simulink subsystem "IMUSensor"  (R2023b)
settings: Solver=VariableStepAuto  StartTime=0.0  StopTime=10.0  RelTol=1e-3
libraries: vehdynlibsens x1
settings Model: Creator=The MathWorks, Inc.  LastModifiedBy=The MathWorks, Inc.

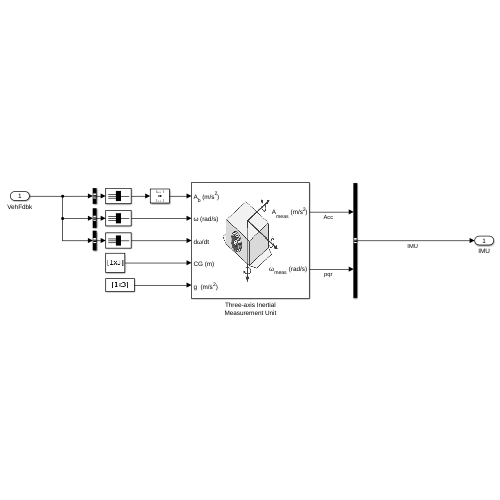
[thumbnail: Simulink's stored preview of the top-level diagram]
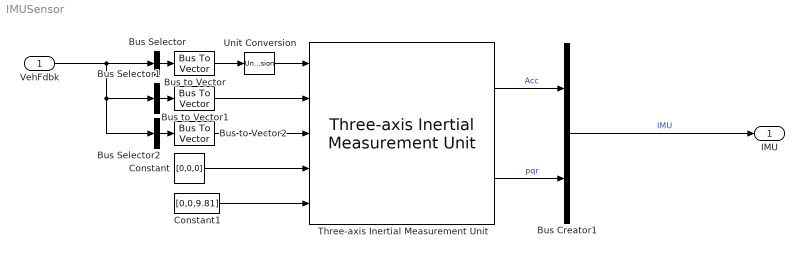
== system IMUSensor ==
  VehFdbk : Inport
  Bus Creator1 : BusCreator  Inputs=2
  Bus Selector : BusSelector  OutputSignals=BdyFrm.Cg.Acc.ax,BdyFrm.Cg.Acc.ay,BdyFrm.Cg.Acc.az  OutputAsBus=on
  Bus Selector1 : BusSelector  OutputSignals=BdyFrm.Cg.AngVel.p,BdyFrm.Cg.AngVel.q,BdyFrm.Cg.AngVel.r  OutputAsBus=on
  Bus Selector2 : BusSelector  OutputSignals=BdyFrm.Cg.AngAcc.pdot,BdyFrm.Cg.AngAcc.qdot,BdyFrm.Cg.AngAcc.rdot  OutputAsBus=on
  Bus to Vector : BusToVector
  Bus to Vector1 : BusToVector
  Bus to Vector2 : BusToVector
  Constant : Constant  Value=[0,0,0]
  Constant1 : Constant  Value=[0,0,9.81]
  Three-axis Inertial Measurement Unit : vehdynlibsens/Three-axis Inertial Measurement Unit  units=Metric (MKS)  imu=[0 0 0]  i_Ts=0  dtype_a=off  w_a=190  z_a=0.707  a_sf_cc=[1 0 0; 0 1 0; 0 0 1]  a_bias=[0 0 0]  a_sat="[-inf  -inf  -inf  inf inf inf]"  dtype_g=off  w_g=190  z_g=0.707  g_sf_cc=[1 0 0; 0 1 0; 0 0 1]  g_bias=[0 0 0]  g_sens=[0 0 0]  g_sat="[-inf  -inf  -inf  inf inf inf]"  i_rand=on  i_seeds=[23093 23094 23095 23096 23097 23098]  i_pow=[0.001 0.001 0.001 0.0001 0.0001 0.0001]  aMode=2
  Unit Conversion : UnitConversion
  IMU : Outport
  wires:
  Unit Conversion/1 -> Three-axis Inertial Measurement Unit/1
  Three-axis Inertial Measurement Unit/2 -> Bus Creator1/2  "pqr"
  Constant/1 -> Three-axis Inertial Measurement Unit/4
  Bus Selector2/1 -> Bus to Vector2/1
  Bus Creator1/1 -> IMU/1  "IMU"
  Three-axis Inertial Measurement Unit/1 -> Bus Creator1/1  "Acc"
  Bus to Vector2/1 -> Three-axis Inertial Measurement Unit/3
  Bus Selector/1 -> Bus to Vector/1
  Bus to Vector1/1 -> Three-axis Inertial Measurement Unit/2
  Bus Selector1/1 -> Bus to Vector1/1
  Bus to Vector/1 -> Unit Conversion/1
  Constant1/1 -> Three-axis Inertial Measurement Unit/5
  VehFdbk/1 -> Bus Selector/1, Bus Selector1/1, Bus Selector2/1
